simulink model "Single_Standalone_Module"  (R2019b)
settings: Solver=VariableStepAuto  StartTime=0.0  StopTime=1  RelTol=1e-3
libraries: powerlib x30, ac_grid_connnected x6, powerlib_meascontrol x4, Power_Electronic_Lab_Controllers x3, Control_Signal_Sources x1
settings Model: Creator=mehdi  LastModifiedBy=mehdi

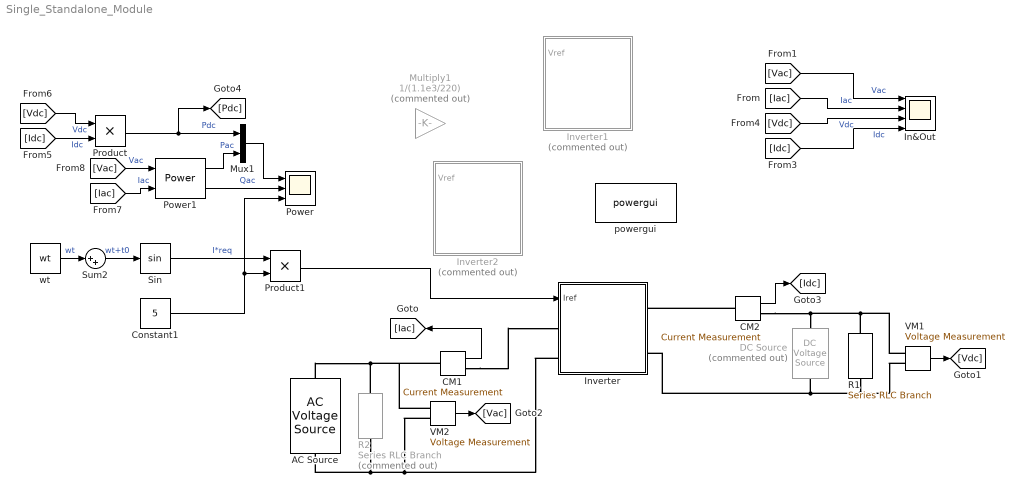
== system Single_Standalone_Module ==
  AC Source : powerlib/Electrical Sources/AC Voltage Source  Amplitude=220*sqrt(2)  Phase=0  Frequency=50  SampleTime=0  Measurements=None  BusType=swing  Pref=10e3  Qref=0  Qmin=-inf  Qmax=+inf
      settings: SourceProductName=Simscape Electrical
  CM1 : powerlib/Measurements/Current Measurement  PhasorSimulation=off  OutputType=Complex  PSBequivalent=0
      settings: SourceProductName=Simscape Electrical
  CM2 : powerlib/Measurements/Current Measurement  PhasorSimulation=off  OutputType=Complex  PSBequivalent=0
      settings: SourceProductName=Simscape Electrical
  Constant1 : Constant  Value=5
  DC Source : powerlib/Electrical Sources/DC Voltage Source  Commented=on  Amplitude=300  Measurements=None
      settings: SourceProductName=Simscape Electrical
  In&Out : Scope  NumInputPorts=4
  Inverter : Subsystem  mask{Pnom=1.1e3, Vnom=400, DC_Vol=600, DC_Cap=2*470e-6, is_cascaded=off, module=2, phase=3, f=50, fsw=10e3, mod_dom=[-1 1], mod_phs=90, input_type=Actaul, filter_type=LCL, L1=0.0089072, r1=0, Cf=1.0942e-06, Rf=42.5424, L2=0.0025465, r2=0, advance_designer=off, dVmax=0.05, dImax=0.5, des_type=dep. Ka, ka=0.1, r=0.1, fres=3419.0493, PR_P=0.1, PR_R=0.5, DC_Init=0, DC_Cap_ESR=0, start_time=0, PR_Scope_En=on, CG=1}
      mask prompts: Pnom "Nominal Power (W)"; Vnom "Nominal Voltage (V)"; DC_Vol "DC Link Voltage (V)"; DC_Cap "Capacitor (F)"; is_cascaded "Cascaded"; module "Number of modules in each phase"; phase "Number of Phases"; f "Found. Frequency (Hz)"; fsw "Switching Frequency (Hz)"; mod_dom "Modulator Domain [min MAX]"; mod_phs "Modulator Phase (Deg)"; input_type "Input Type"; filter_type "Filter Type"; L1 "Converter Side Ind (H)"; r1 "Converter Side Res (Ohm)"; Cf "Filter Capacitor (F)"; Rf "Filter Resistor (Ohm)"; L2 "Grid Side Ind (H)"; r2 "Grid Side Res (Ohm)"; advance_designer "Advance Designer"; dVmax "Max Accepted Voltage Variation"; dImax "Max Accepted Current Variation"; des_type "Designer Type"; fres "Resonant Freq."; PR_P "P"; PR_R "R"; DC_Init "DC Link Init (V)"; DC_Cap_ESR "DC Llink Cap ESR (Ohm)"; start_time "Start Time (s)"; PR_Scope_En "PR Controller Scope"; CG "Current Gain"
      mask Callback Pnom:
      | typ = get_param(gcb, 'input_type');
      | Pnom = str2num(get_param(gcb, 'Pnom'));
      | Vnom = str2num(get_param(gcb, 'Vnom'));
      | 
      | if strcmp(typ, 'Normalized')
      |     Inom = Pnom / Vnom ;
      |     set_param(gcb, 'CG', num2str(1 / Inom));
      | else
      |     set_param(gcb, 'CG', num2str(1));
      | end
      mask Callback Vnom:
      | typ = get_param(gcb, 'input_type');
      | Pnom = str2num(get_param(gcb, 'Pnom'));
      | Vnom = str2num(get_param(gcb, 'Vnom'));
      | 
      | if strcmp(typ, 'Normalized')
      |     Inom = Pnom / Vnom ;
      |     set_param(gcb, 'CG', num2str(1 / Inom));
      | else
      |     set_param(gcb, 'CG', num2str(1));
      | end
      mask Callback is_cascaded:
      | cas = get_param(gcb, 'is_cascaded');
      | mask = Simulink.Mask.get(gcb);
      | module = mask.getParameter('module');
      | phase  = mask.getParameter('phase');
      | 
      | if strcmp(cas, 'on')
      |     module.Visible = 'on';
      |     phase.Visible  = 'on';
      | 
      | else
      |     module.Visible = 'off';
      |     phase.Visible  = 'off';
      | 
      | end
      mask TypeOptions input_type: Actaul | Normalized
      mask Callback input_type:
      | typ = get_param(gcb, 'input_type');
      | Pnom = str2num(get_param(gcb, 'Pnom'));
      | Vnom = str2num(get_param(gcb, 'Vnom'));
      | 
      | if strcmp(typ, 'Normalized')
      |     Inom = Pnom / Vnom ;
      |     set_param(gcb, 'CG', num2str(1 / Inom));
      | else
      |     set_param(gcb, 'CG', num2str(1));
      | end
      mask TypeOptions filter_type: L | LC | LCL | LCL_imp
      mask Callback filter_type:
      | typ = get_param(gcb, 'filter_type');
      | mask = Simulink.Mask.get(gcb);
      | hL1 = mask.getParameter('L1');
      | hL2 = mask.getParameter('L2');
      | hCf = mask.getParameter('Cf');
      | hRf = mask.getParameter('Rf');
      | hr1 = mask.getParameter('r1');
      | hr2 = mask.getParameter('r2');
      | hKa = mask.getParameter('ka');
      | hR  = mask.getParameter('r');
      | hFr = mask.getParameter('fres');
      | hDT = mask.getParameter('des_type');
      | 
      | switch typ
      |     case 'L'
      |         hL2.Visible = 'off';
      |         hr2.Visible = 'off';
      |         hCf.Visible = 'off';
      |         hRf.Visible = 'off';
      |         hFr.Visible = 'off';
      |         hDT.Visible = 'off';
      |         hKa.Visible = 'off';
      |         hR.Visible  = 'off';
      | 
      |     case 'LC'
      |         hL2.Visible = 'off';
      |         hr2.Visible = 'off';
      |         hCf.Visible = 'on';
      |         hRf.Visible = 'on';
      |         hFr.Visible = 'on';
      |         hDT.Visible = 'off';
      |         hKa.Visible = 'off';
      |         hR.Visible  = 'off';
      | 
      |     case 'LCL'
      |         hL2.Visible = 'on';
      |         hr2.Visible = 'on';
      |         hCf.Visible = 'on';
      |         hRf.Visible = 'on';
      |         hFr.Visible = 'on';
      |         hDT.Visible = 'on';
      |         if strcmp(get_param(gcb, 'des_type'), 'dep. r')
      |             hR.Visible = 'on';
      |             hKa.Visible = 'off';
      |         else
      |             hR.Visible = 'off';
      |             hKa.Visible = 'on';
      |         end
      | end
      mask Callback advance_designer:
      | adv = get_param(gcb, 'advance_designer');
      | mask = Simulink.Mask.get(gcb);
      | dV = mask.getParameter('dVmax');
      | dI = mask.getParameter('dImax');
      | if strcmp(adv, 'on')
      |     dV.Visible = 'on';
      |     dI.Visible = 'on';
      | else
      |     dV.Visible = 'off';
      |     dI.Visible = 'off';
      | end
      mask TypeOptions des_type: dep. Ka | dep. r
      mask Callback des_type:
      | dep = get_param(gcb, 'des_type');
      | mask = Simulink.Mask.get(gcb);
      | ka = mask.getParameter('ka');
      | r  = mask.getParameter('r');
      | 
      | if strcmp(dep, 'dep. Ka')
      |     ka.Visible = 'on';
      |     r.Visible = 'off';
      | 
      | else
      |     ka.Visible = 'off';
      |     r.Visible = 'on';
      | 
      | end
      mask Callback PR_Scope_En:
      | enable = get_param(gcb, 'PR_Scope_En');
      | scope = getSimulinkBlockHandle(strjoin({gcb, 'PR'}, '/'));
      | 
      | if strcmp(enable, 'on')
      |     set(scope, 'Commented', 'off')
      | else
      |     set(scope, 'Commented', 'on')
      | end
      mask DialogControl Container7 Prompt: Basic
      mask DialogControl Container10 Prompt: Filter
      mask DialogControl Container16 Prompt: Filter Elements
      mask DialogControl cal Prompt: Calculator
      mask DialogControl cal Callback:
      | powericon('SinglePhaseLCLFIlterDesigner', 'calculator')
      | %powericon('ThreePhaseVSIwithLCL_CallBack', 'LCLFilterCalculator');
      mask DialogControl des Prompt: Designer
      mask DialogControl des Callback:
      | powericon('SinglePhaseLCLFIlterDesigner', 'desinger')
      | %powericon('ThreePhaseVSIwithLCL_CallBack', 'LCLFilterDesigner');
      mask DialogControl Container13 Prompt: Control & Simulation
      mask DialogControl Container14 Prompt: Control Parameters
      mask DialogControl Container17 Prompt: Initiat Values
      mask DialogControl Container18 Prompt: Simulation Controll
      mask DialogControl Container11 Prompt: Hidden Items
      mask Display: disp('Single\nPhase\nModule')
  Inverter1 : Subsystem  Commented=on  mask{Pnom=1.1e3, Vnom=230, DC_Vol=400, DC_Cap=470e-6, is_cascaded=off, module=2, phase=3, f=50, fsw=10e3, mod_dom=[-1 1], mod_phs=90, start_time=0, input_type=Actaul, L1=0.005914, L2=0.00084193, Cf=3.3095e-06, Rf=14.923, advance_designer=on, dVmax=0.05, dImax=0.5, des_type=dep. Ka, ka=0.1, r=0, fres=3222.5943, PR_P=0, PR_R=0}
      mask prompts: Pnom "Nominal Power (W)"; Vnom "Nominal Voltage (V)"; DC_Vol "DC Link Voltage (V)"; DC_Cap "Capacitor (F)"; is_cascaded "Cascaded"; module "Number of modules in each phase"; phase "Number of Phases"; f "Found. Frequency (Hz)"; fsw "Switching Frequency (Hz)"; mod_dom "Modulator Domain [min MAX]"; mod_phs "Modulator Phase (Deg)"; start_time "Start Time (s)"; input_type "Input Type"; L1 "Converter Side Ind (H)"; L2 "Grid Side Ind (H)"; Cf "Filter Capacitor (F)"; Rf "Filter Resistor (Ohm)"; advance_designer "Advance Designer"; dVmax "Max Accepted Voltage Variation"; dImax "Max Accepted Current Variation"; des_type "Designer Type"; fres "Resonant Freq."; PR_P "Prop Gain"; PR_R "Reso Gain"
      mask Callback is_cascaded:
      | cas = get_param(gcb, 'is_cascaded');
      | mask = Simulink.Mask.get(gcb);
      | module = mask.getParameter('module');
      | phase  = mask.getParameter('phase');
      | 
      | if strcmp(cas, 'on')
      |     module.Visible = 'on';
      |     phase.Visible  = 'on';
      | 
      | else
      |     module.Visible = 'off';
      |     phase.Visible  = 'off';
      | 
      | end
      mask TypeOptions input_type: Actaul | Normalized
      mask Callback advance_designer:
      | adv = get_param(gcb, 'advance_designer');
      | mask = Simulink.Mask.get(gcb);
      | dV = mask.getParameter('dVmax');
      | dI = mask.getParameter('dImax');
      | if strcmp(adv, 'on')
      |     dV.Visible = 'on';
      |     dI.Visible = 'on';
      | else
      |     dV.Visible = 'off';
      |     dI.Visible = 'off';
      | end
      mask TypeOptions des_type: dep. Ka | dep. r
      mask Callback des_type:
      | dep = get_param(gcb, 'des_type');
      | mask = Simulink.Mask.get(gcb);
      | ka = mask.getParameter('ka');
      | r  = mask.getParameter('r');
      | 
      | if strcmp(dep, 'dep. Ka')
      |     ka.Visible = 'on';
      |     r.Visible = 'off';
      | 
      | else
      |     ka.Visible = 'off';
      |     r.Visible = 'on';
      | 
      | end
      mask DialogControl Container7 Prompt: Basic
      mask DialogControl Container14 Prompt: Switching
      mask DialogControl Container10 Prompt: Filter
      mask DialogControl cal Prompt: Calculator
      mask DialogControl cal Callback: powericon('SinglePhaseLCLFIlterDesigner', 'calculator')
      mask DialogControl des Prompt: Designer
      mask DialogControl des Callback: powericon('SinglePhaseLCLFIlterDesigner', 'designer')
      mask DialogControl Container13 Prompt: Controller
      mask Display: disp('Inverter')
  Inverter2 : Subsystem  Commented=on  mask{Pnom=1.1e3, Vnom=230, DC_Vol=400, DC_Cap=470e-6, is_cascaded=on, module=2, phase=3, f=50, fsw=10e3, mod_dom=[-1 1], mod_phs=90, start_time=0, input_type=Actaul, L1=0.0089072, L2=0.00084193, Cf=3.3095e-06, Rf=11.7134, advance_designer=on, dVmax=0.05, dImax=0.5, des_type=dep. Ka, ka=0.1, r=0, fres=4105.6226, PR_P=0, PR_R=0, DC_Init=0, DC_Cap_ESR=0}
      mask prompts: Pnom "Nominal Power (W)"; Vnom "Nominal Voltage (V)"; DC_Vol "DC Link Voltage (V)"; DC_Cap "Capacitor (F)"; is_cascaded "Cascaded"; module "Number of modules in each phase"; phase "Number of Phases"; f "Found. Frequency (Hz)"; fsw "Switching Frequency (Hz)"; mod_dom "Modulator Domain [min MAX]"; mod_phs "Modulator Phase (Deg)"; start_time "Start Time (s)"; input_type "Input Type"; L1 "Converter Side Ind (H)"; L2 "Grid Side Ind (H)"; Cf "Filter Capacitor (F)"; Rf "Filter Resistor (Ohm)"; advance_designer "Advance Designer"; dVmax "Max Accepted Voltage Variation"; dImax "Max Accepted Current Variation"; des_type "Designer Type"; fres "Resonant Freq."; PR_P "Prop Gain"; PR_R "Reso Gain"; DC_Init "DC Link Init (V)"; DC_Cap_ESR "DC Llink Cap ESR (Ohm)"
      mask Callback is_cascaded:
      | cas = get_param(gcb, 'is_cascaded');
      | mask = Simulink.Mask.get(gcb);
      | module = mask.getParameter('module');
      | phase  = mask.getParameter('phase');
      | 
      | if strcmp(cas, 'on')
      |     module.Visible = 'on';
      |     phase.Visible  = 'on';
      | 
      | else
      |     module.Visible = 'off';
      |     phase.Visible  = 'off';
      | 
      | end
      mask TypeOptions input_type: Actaul | Normalized
      mask Callback advance_designer:
      | adv = get_param(gcb, 'advance_designer');
      | mask = Simulink.Mask.get(gcb);
      | dV = mask.getParameter('dVmax');
      | dI = mask.getParameter('dImax');
      | if strcmp(adv, 'on')
      |     dV.Visible = 'on';
      |     dI.Visible = 'on';
      | else
      |     dV.Visible = 'off';
      |     dI.Visible = 'off';
      | end
      mask TypeOptions des_type: dep. Ka | dep. r
      mask Callback des_type:
      | dep = get_param(gcb, 'des_type');
      | mask = Simulink.Mask.get(gcb);
      | ka = mask.getParameter('ka');
      | r  = mask.getParameter('r');
      | 
      | if strcmp(dep, 'dep. Ka')
      |     ka.Visible = 'on';
      |     r.Visible = 'off';
      | 
      | else
      |     ka.Visible = 'off';
      |     r.Visible = 'on';
      | 
      | end
      mask DialogControl Container7 Prompt: Basic
      mask DialogControl Container10 Prompt: Filter
      mask DialogControl cal Prompt: Calculator
      mask DialogControl cal Callback:
      | %powericon('SinglePhaseLCLFIlterDesigner', 'calculator')
      | powericon('ThreePhaseVSIwithLCL_CallBack', 'LCLFilterCalculator');
      mask DialogControl des Prompt: Designer
      mask DialogControl des Callback:
      | %powericon('SinglePhaseLCLFIlterDesigner', 'designer')
      | powericon('ThreePhaseVSIwithLCL_CallBack', 'LCLFilterDesigner');
      mask DialogControl Container13 Prompt: Controller
      mask Display: disp('Inverter')
  Multiply1 : Gain  Commented=on  Gain=1/(1.1e3/220)
  Mux1 : Mux  Inputs=2
  Power : Scope  NumInputPorts=3
  Power1 : powerlib_meascontrol/Measurements/Power  Freq=50  Vinit=[1, 0]  Iinit=[1, 0]  Ts=0
      settings: SourceProductName=Simscape Electrical
  Product : Product
  Product1 : Product
  R1 : powerlib/Elements/Series RLC Branch  LConnTagsString=__new0  RConnTagsString=__new0  BranchType=R  Resistance=82  Inductance=1e-3  SetiL0=off  InitialCurrent=0  Capacitance=1e-6  Setx0=off  InitialVoltage=0  Measurements=None
      settings: SourceProductName=Simscape Electrical
  R2 : powerlib/Elements/Series RLC Branch  Commented=on  LConnTagsString=__new0  RConnTagsString=__new0  BranchType=R  Resistance=40  Inductance=1e-3  SetiL0=off  InitialCurrent=0  Capacitance=1e-6  Setx0=off  InitialVoltage=0  Measurements=None
      settings: SourceProductName=Simscape Electrical
  Sin : Trigonometry
  Sum2 : Sum  Inputs=|++
  VM1 : powerlib/Measurements/Voltage Measurement  PhasorSimulation=off  OutputType=Complex  PSBequivalent=0
      settings: SourceProductName=Simscape Electrical
  VM2 : powerlib/Measurements/Voltage Measurement  PhasorSimulation=off  OutputType=Complex  PSBequivalent=0
      settings: SourceProductName=Simscape Electrical
  powergui : powerlib/powergui  Priority=1  SimulationMode=Continuous  SampleTime=50e-6  frequency=60  Iterations=50  frequencyindice=50  Pbase=100e6  ErrMax=1e-4  UnitsV=kV  UnitsW=MW  buscounter=0  FunctionMessages=off  echomessages=off  EnableUseOfTLC=off  CurrentSourceSwitches=off  DisableSnubberDevices=off  DisableRonSwitches=off  DisableVfSwitches=off  DisplayEquations=off  AutomaticDiscreteSolvers=off  SolverType=Tustin/Backward Euler (TBE)  Interpol=off  ExternalGateDelay=off  methode=off  Ts=100  x0status=blocks  SPID=on  SwTol=0  HookPort=off  NonlinearTolerance=1e-4  nMaxIteration=100  ContinueOnMaxIteration=off  RestoreLinks=warning  ResistiveCurrentMeasurement=off  Frange=[0:2:500]  Ylog=off  Xlog=on  ShowGrid=off  save=off  variable=ZData  structure=0  ZoomFFT=off  StartTime=0.0  cycles=1  DisplayStyle=1  fundamental=60  FreqAxis=off  MaxFrequency=1000  frequencyindicesteady=1  RmsSteady=1  display=off
      settings: SourceProductName=Simscape Electrical
  wt : Control_Signal_Sources/wt  f=100*pi  R=[-pi pi]
      settings: SourceProductName=Power Electronic Lab
  wires:
  CM1/1 -> [Iac]
  VM1/1 -> [Vdc]
  [Iac] -> In&Out/2  "Iac"
  VM2/1 -> [Vac]
  [Vac] -> In&Out/1  "Vac"
  CM2/1 -> [Idc]
  [Idc] -> In&Out/4  "Idc"
  [Vdc] -> In&Out/3  "Vdc"
  [Vdc] -> Product/1  "Vdc"
  [Idc] -> Product/2  "Idc"
  Sum2/1 -> Sin/1  "wt+t0"
  wt/1 -> Sum2/1  "wt"
  Power1/1 -> Mux1/2  "Pac"
  Mux1/1 -> Power/1
  [Vac] -> Power1/1  "Vac"
  [Iac] -> Power1/2  "Iac"
  Power1/2 -> Power/2  "Qac"
  Product/1 -> [Pdc], Mux1/1  "Pdc"
  Sin/1 -> Product1/1  "I*req"
  Product1/1 -> Inverter/1(Iref)
  Constant1/1 -> Product1/2, Power/3
  connections:
  R1/LConn1 -- VM1/LConn1 -- CM2/RConn1 -- DC Source/RConn1
  AC Source/RConn1 -- CM1/LConn1 -- VM2/LConn1 -- R2/LConn1
  VM2/LConn2 -- Inverter/LConn2 -- R2/RConn1 -- AC Source/LConn1
  VM1/LConn2 -- R1/RConn1 -- Inverter/RConn2 -- DC Source/LConn1
  CM2/LConn1 -- Inverter/RConn1
  CM1/RConn1 -- Inverter/LConn1

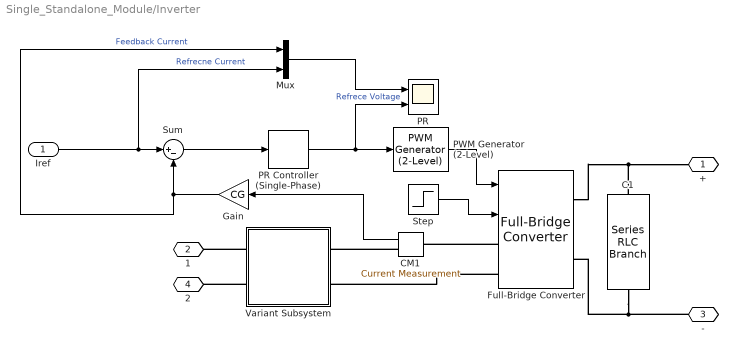
== system Single_Standalone_Module/Inverter ==
  Iref : Inport
  C1 : powerlib/Elements/Series RLC Branch  LConnTagsString=__new0  RConnTagsString=__new0  BranchType=RC  Resistance=DC_Cap_ESR  Inductance=0  SetiL0=off  InitialCurrent=0  Capacitance=DC_Cap  Setx0=on  InitialVoltage=DC_Init  Measurements=None
      settings: SourceProductName=Simscape Electrical
  CM1 : powerlib/Measurements/Current Measurement  PhasorSimulation=off  OutputType=Complex  PSBequivalent=0
      settings: SourceProductName=Simscape Electrical
  Full-Bridge Converter : powerlib/Power Electronics/Full-Bridge Converter  ModelType=Switching devices  Ron=1e-3  Rs=1e6  Cs=inf  Vforward=[0,0]  Ron_Diode=1e-3  Rs_Diode=1e6  Cs_Diode=inf  Vf_Diode=1e-3  Rs_CurrentSource=inf
      settings: SourceProductName=Simscape Electrical  SourceProductBaseCode=PS
  Gain : Gain  Gain=CG
  Mux : Mux  Inputs=2
  PR : Scope  NumInputPorts=2
  PR Controller (Single-Phase) : Power_Electronic_Lab_Controllers/PR Controller (Single-Phase)  Kp=PR_P  Kr=PR_R  w0=2*pi*f
      settings: SourceProductName=Power Electronic Lab
  PWM Generator (2-Level) : powerlib_meascontrol/Pulse & Signal Generators/PWM Generator (2-Level)  ModulatorType=Single-phase full-bridge (4 pulses)  ModulatorMode=Unsynchronized  Fc=fsw  Pc=mod_phs  nF=27  MinMax=mod_dom  SamplingTechnique=Natural  ModulatingSignals=off  m=0.8  Freq=60  Phase=0  Ts=0  ShowCarrierOutport=off
  Step : Step  Time=start_time  Before=1  After=0  SampleTime=0
  Sum : Sum  Inputs=|+-
  Variant Subsystem : Subsystem  VariantControlMode=Label  Variant=on  LabelModeActiveChoice=LCL_imp  mask{tp=filter_type, L1=L1, r1=r1, L2=L2, r2=r2, Cf=Cf, Rf=Rf}
      mask prompts: tp "Filter Type"
      mask Callback tp:
      | tp = get_param(gcb, 'tp');
      | 
      | switch tp
      |     case 'L'
      |         set_param(gcb, 'LabelModeActivechoice', 'L')
      | 
      |     case 'LC'
      |         set_param(gcb, 'LabelModeActivechoice', 'LC')
      | 
      |     case 'LCL'
      |         set_param(gcb, 'LabelModeActivechoice', 'LCL')
      | 
      |     case 'Devided LCL'
      |         set_param(gcb, 'LabelModeActivechoice', 'LCL_imp')
      | end
  + : PMIOPort  Side=Right
  1 : PMIOPort  Port=2  Side=Left
  - : PMIOPort  Port=3  Side=Right
  2 : PMIOPort  Port=4  Side=Left
  wires:
  PWM Generator (2-Level)/1 -> Full-Bridge Converter/1
  Step/1 -> Full-Bridge Converter/2
  Sum/1 -> PR Controller (Single-Phase)/1
  PR Controller (Single-Phase)/1 -> PR/2, PWM Generator (2-Level)/1  "Refrece Voltage"
  Iref/1 -> Mux/2, Sum/1  "Refrecne Current"
  Mux/1 -> PR/1
  Gain/1 -> Mux/1, Sum/2  "Feedback Current"
  CM1/1 -> Gain/1
  connections:
  Full-Bridge Converter/RConn1 -- C1/LConn1 -- +/RConn1
  -/RConn1 -- C1/RConn1 -- Full-Bridge Converter/RConn2
  Variant Subsystem/RConn2 -- 2/RConn1
  Full-Bridge Converter/LConn2 -- Variant Subsystem/LConn2
  Full-Bridge Converter/LConn1 -- CM1/LConn1
  CM1/RConn1 -- Variant Subsystem/LConn1
  Variant Subsystem/RConn1 -- 1/RConn1

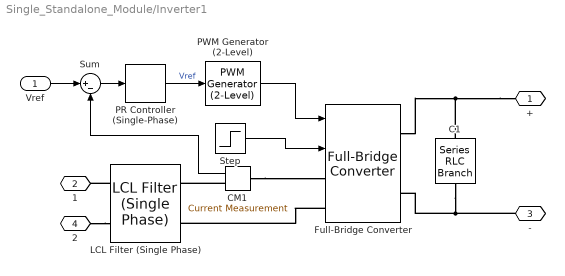
== system Single_Standalone_Module/Inverter1 ==
  Vref : Inport
  C1 : powerlib/Elements/Series RLC Branch  LConnTagsString=__new0  RConnTagsString=__new0  BranchType=C  Resistance=40  Inductance=1e-3  SetiL0=off  InitialCurrent=0  Capacitance=470e-6  Setx0=off  InitialVoltage=0  Measurements=None
      settings: SourceProductName=Simscape Electrical
  CM1 : powerlib/Measurements/Current Measurement  PhasorSimulation=off  OutputType=Complex  PSBequivalent=0
      settings: SourceProductName=Simscape Electrical
  Full-Bridge Converter : powerlib/Power Electronics/Full-Bridge Converter  ModelType=Switching devices  Ron=1e-3  Rs=1e6  Cs=inf  Vforward=[0,0]  Ron_Diode=1e-3  Rs_Diode=1e6  Cs_Diode=inf  Vf_Diode=1e-3  Rs_CurrentSource=inf
      settings: SourceProductName=Simscape Electrical  SourceProductBaseCode=PS
  LCL Filter (Single Phase) : ac_grid_connnected/LCL Filter (Single Phase)  Vn=400  Vdc=600  Sn=1.1e3  f=50  fsw=10e3  L1=0.0089072  L2=0.0025465  Cf=1.0942e-06  Rf=42.5424  advance_designer_ckb=on  dVmax=0.05  dImax=0.5  des_pop=known ka  ka=0.1  r=0  fres=3419.0493
      settings: SourceProductName=Power Electronic Lab
  PR Controller (Single-Phase) : Power_Electronic_Lab_Controllers/PR Controller (Single-Phase)  Kp=0.1  Kr=0.5  w0=100*pi
      settings: SourceProductName=Power Electronic Lab
  PWM Generator (2-Level) : powerlib_meascontrol/Pulse & Signal Generators/PWM Generator (2-Level)  ModulatorType=Single-phase full-bridge (4 pulses)  ModulatorMode=Unsynchronized  Fc=10e3  Pc=90  nF=27  MinMax="[ -1  1 ]"  SamplingTechnique=Natural  ModulatingSignals=off  m=0.8  Freq=60  Phase=0  Ts=0  ShowCarrierOutport=off
  Step : Step  Time=0  Before=1  After=0  SampleTime=0
  Sum : Sum  Inputs=|+-
  + : PMIOPort  Side=Right
  1 : PMIOPort  Port=2  Side=Left
  - : PMIOPort  Port=3  Side=Right
  2 : PMIOPort  Port=4  Side=Left
  wires:
  CM1/1 -> Sum/2
  Vref/1 -> Sum/1
  PR Controller (Single-Phase)/1 -> PWM Generator (2-Level)/1  "Vref"
  Sum/1 -> PR Controller (Single-Phase)/1
  Step/1 -> Full-Bridge Converter/2
  PWM Generator (2-Level)/1 -> Full-Bridge Converter/1
  connections:
  CM1/RConn1 -- LCL Filter (Single Phase)/LConn1
  CM1/LConn1 -- Full-Bridge Converter/LConn1
  Full-Bridge Converter/RConn2 -- C1/RConn1 -- -/RConn1
  +/RConn1 -- C1/LConn1 -- Full-Bridge Converter/RConn1
  Full-Bridge Converter/LConn2 -- LCL Filter (Single Phase)/LConn2
  2/RConn1 -- LCL Filter (Single Phase)/RConn2
  LCL Filter (Single Phase)/RConn1 -- 1/RConn1

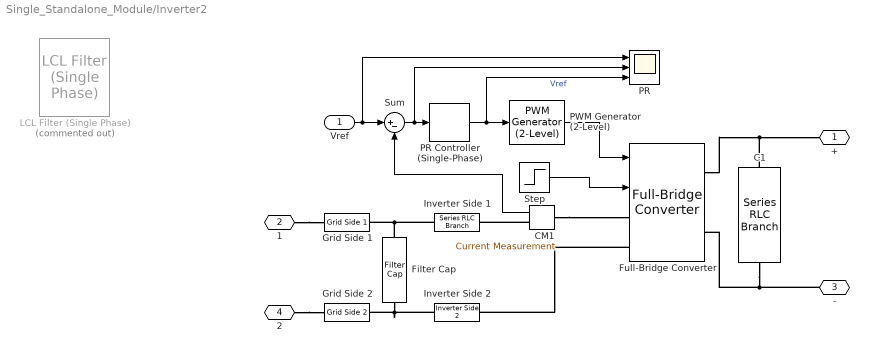
== system Single_Standalone_Module/Inverter2 ==
  Vref : Inport
  C1 : powerlib/Elements/Series RLC Branch  LConnTagsString=__new0  RConnTagsString=__new0  BranchType=RC  Resistance=DC_Cap_ESR  Inductance=0  SetiL0=off  InitialCurrent=0  Capacitance=DC_Cap  Setx0=on  InitialVoltage=DC_Init  Measurements=None
      settings: SourceProductName=Simscape Electrical
  CM1 : powerlib/Measurements/Current Measurement  PhasorSimulation=off  OutputType=Complex  PSBequivalent=0
      settings: SourceProductName=Simscape Electrical
  Filter Cap : ac_grid_connnected/LCL Filter (Single Phase)/Filter Cap  LConnTagsString=__new0  RConnTagsString=__new0  BranchType=RC  Resistance=Rf  Inductance=L2  SetiL0=off  InitialCurrent=0  Capacitance=Cf  Setx0=off  InitialVoltage=0  Measurements=None
      settings: SourceProductName=Power Electronic Lab
  Full-Bridge Converter : powerlib/Power Electronics/Full-Bridge Converter  ModelType=Switching devices  Ron=1e-3  Rs=1e6  Cs=inf  Vforward=[0,0]  Ron_Diode=1e-3  Rs_Diode=1e6  Cs_Diode=inf  Vf_Diode=1e-3  Rs_CurrentSource=inf
      settings: SourceProductName=Simscape Electrical  SourceProductBaseCode=PS
  Grid Side 1 : ac_grid_connnected/LCL Filter (Single Phase)/Grid Side 1  LConnTagsString=__new0  RConnTagsString=__new0  BranchType=L  Resistance=1  Inductance=L2/2  SetiL0=off  InitialCurrent=0  Capacitance=1e-6  Setx0=off  InitialVoltage=0  Measurements=None
      settings: SourceProductName=Power Electronic Lab
  Grid Side 2 : ac_grid_connnected/LCL Filter (Single Phase)/Grid Side 2  LConnTagsString=__new0  RConnTagsString=__new0  BranchType=L  Resistance=1  Inductance=L2/2  SetiL0=off  InitialCurrent=0  Capacitance=1e-6  Setx0=off  InitialVoltage=0  Measurements=None
      settings: SourceProductName=Power Electronic Lab
  Inverter Side 1 : powerlib/Elements/Series RLC Branch  LConnTagsString=__new0  RConnTagsString=__new0  BranchType=L  Resistance=1  Inductance=L1/2  SetiL0=off  InitialCurrent=0  Capacitance=1e-6  Setx0=off  InitialVoltage=0  Measurements=None
      settings: SourceProductName=Simscape Electrical
  Inverter Side 2 : ac_grid_connnected/LCL Filter (Single Phase)/Inverter Side 2  LConnTagsString=__new0  RConnTagsString=__new0  BranchType=L  Resistance=1  Inductance=L1/2  SetiL0=off  InitialCurrent=0  Capacitance=1e-6  Setx0=off  InitialVoltage=0  Measurements=None
      settings: SourceProductName=Power Electronic Lab
  LCL Filter (Single Phase) : ac_grid_connnected/LCL Filter (Single Phase)  Commented=on  Vn=400  Vdc=600  Sn=1.1e3  f=50  fsw=10e3  L1=L1  L2=L2  Cf=Cf  Rf=Rf  advance_designer_ckb=on  dVmax=0.05  dImax=0.5  des_pop=known ka  ka=0.1  r=0  fres=3419.0493
      settings: SourceProductName=Power Electronic Lab
  PR : Scope  NumInputPorts=3
  PR Controller (Single-Phase) : Power_Electronic_Lab_Controllers/PR Controller (Single-Phase)  Kp=0.1  Kr=0.5  w0=100*pi
      settings: SourceProductName=Power Electronic Lab
  PWM Generator (2-Level) : powerlib_meascontrol/Pulse & Signal Generators/PWM Generator (2-Level)  ModulatorType=Single-phase full-bridge (4 pulses)  ModulatorMode=Unsynchronized  Fc=fsw  Pc=mod_phs  nF=27  MinMax=mod_dom  SamplingTechnique=Natural  ModulatingSignals=off  m=0.8  Freq=60  Phase=0  Ts=0  ShowCarrierOutport=off
  Step : Step  Time=start_time  Before=1  After=0  SampleTime=0
  Sum : Sum  Inputs=|+-
  + : PMIOPort  Side=Right
  1 : PMIOPort  Port=2  Side=Left
  - : PMIOPort  Port=3  Side=Right
  2 : PMIOPort  Port=4  Side=Left
  wires:
  CM1/1 -> Sum/2
  Vref/1 -> Sum/1, PR/1
  PR Controller (Single-Phase)/1 -> PWM Generator (2-Level)/1, PR/3  "Vref"
  Sum/1 -> PR Controller (Single-Phase)/1, PR/2
  Step/1 -> Full-Bridge Converter/2
  PWM Generator (2-Level)/1 -> Full-Bridge Converter/1
  connections:
  Full-Bridge Converter/LConn2 -- Inverter Side 2/RConn1
  CM1/RConn1 -- Inverter Side 1/LConn1
  Grid Side 2/RConn1 -- Filter Cap/RConn1 -- Inverter Side 2/LConn1
  Grid Side 1/LConn1 -- Filter Cap/LConn1 -- Inverter Side 1/RConn1
  1/RConn1 -- Grid Side 1/RConn1
  2/RConn1 -- Grid Side 2/LConn1
  CM1/LConn1 -- Full-Bridge Converter/LConn1
  Full-Bridge Converter/RConn2 -- C1/RConn1 -- -/RConn1
  C1/LConn1 -- Full-Bridge Converter/RConn1 -- +/RConn1

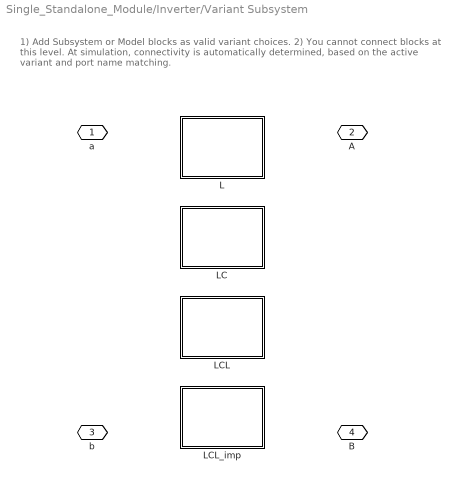
== system Single_Standalone_Module/Inverter/Variant Subsystem ==
  note: 1) Add Subsystem or Model blocks as valid variant choices.
      | 2) You cannot connect blocks at this level. At simulation, connectivity is automatically
      | determined, based on the active variant and port name matching.
  L : Subsystem  VariantControl=L
  LC : Subsystem  VariantControl=LC
  LCL : Subsystem  VariantControl=LCL
  LCL_imp : Subsystem  VariantControl=LCL_imp
  a : PMIOPort  Side=Right
  A : PMIOPort  Port=2  Side=Left
  b : PMIOPort  Port=3  Side=Right
  B : PMIOPort  Port=4  Side=Left

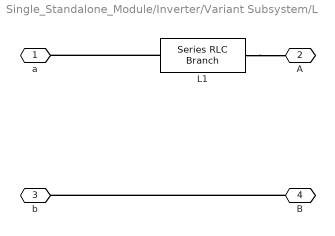
== system Single_Standalone_Module/Inverter/Variant Subsystem/L ==
  L1 : powerlib/Elements/Series RLC Branch  LConnTagsString=__new0  RConnTagsString=__new0  BranchType=RL  Resistance=r1  Inductance=L1  SetiL0=off  InitialCurrent=0  Capacitance=1e-6  Setx0=off  InitialVoltage=0  Measurements=None
      settings: SourceProductName=Simscape Electrical
  a : PMIOPort  Side=Right
  A : PMIOPort  Port=2  Side=Left
  b : PMIOPort  Port=3  Side=Right
  B : PMIOPort  Port=4  Side=Left
  connections:
  B/RConn1 -- b/RConn1
  L1/RConn1 -- a/RConn1
  L1/LConn1 -- A/RConn1

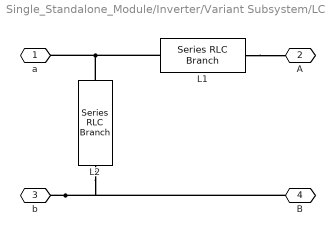
== system Single_Standalone_Module/Inverter/Variant Subsystem/LC ==
  L1 : powerlib/Elements/Series RLC Branch  LConnTagsString=__new0  RConnTagsString=__new0  BranchType=RL  Resistance=r1  Inductance=L1  SetiL0=off  InitialCurrent=0  Capacitance=1e-6  Setx0=off  InitialVoltage=0  Measurements=None
      settings: SourceProductName=Simscape Electrical
  L2 : powerlib/Elements/Series RLC Branch  LConnTagsString=__new0  RConnTagsString=__new0  BranchType=RC  Resistance=Rf  Inductance=L1  SetiL0=off  InitialCurrent=0  Capacitance=Cf  Setx0=off  InitialVoltage=0  Measurements=None
      settings: SourceProductName=Simscape Electrical
  a : PMIOPort  Side=Right
  A : PMIOPort  Port=2  Side=Left
  b : PMIOPort  Port=3  Side=Right
  B : PMIOPort  Port=4  Side=Left
  connections:
  L1/LConn1 -- A/RConn1
  L2/LConn1 -- L1/RConn1 -- a/RConn1
  b/RConn1 -- L2/RConn1 -- B/RConn1

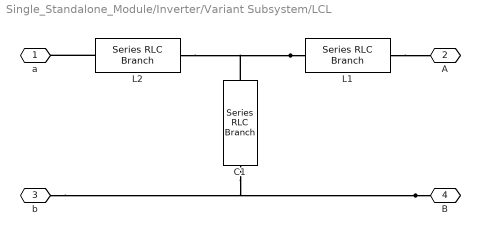
== system Single_Standalone_Module/Inverter/Variant Subsystem/LCL ==
  C1 : powerlib/Elements/Series RLC Branch  LConnTagsString=__new0  RConnTagsString=__new0  BranchType=RC  Resistance=Rf  Inductance=L1  SetiL0=off  InitialCurrent=0  Capacitance=Cf  Setx0=off  InitialVoltage=0  Measurements=None
      settings: SourceProductName=Simscape Electrical
  L1 : powerlib/Elements/Series RLC Branch  LConnTagsString=__new0  RConnTagsString=__new0  BranchType=RL  Resistance=r1  Inductance=L1  SetiL0=off  InitialCurrent=0  Capacitance=1e-6  Setx0=off  InitialVoltage=0  Measurements=None
      settings: SourceProductName=Simscape Electrical
  L2 : powerlib/Elements/Series RLC Branch  LConnTagsString=__new0  RConnTagsString=__new0  BranchType=RL  Resistance=r2  Inductance=L2  SetiL0=off  InitialCurrent=0  Capacitance=1e-6  Setx0=off  InitialVoltage=0  Measurements=None
      settings: SourceProductName=Simscape Electrical
  a : PMIOPort  Side=Right
  A : PMIOPort  Port=2  Side=Left
  b : PMIOPort  Port=3  Side=Right
  B : PMIOPort  Port=4  Side=Left
  connections:
  B/RConn1 -- C1/RConn1 -- b/RConn1
  L1/RConn1 -- C1/LConn1 -- L2/LConn1
  L1/LConn1 -- A/RConn1
  L2/RConn1 -- a/RConn1

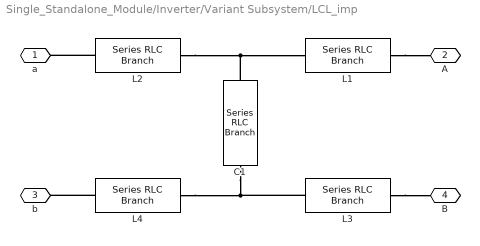
== system Single_Standalone_Module/Inverter/Variant Subsystem/LCL_imp ==
  C1 : powerlib/Elements/Series RLC Branch  LConnTagsString=__new0  RConnTagsString=__new0  BranchType=RC  Resistance=Rf  Inductance=L1  SetiL0=off  InitialCurrent=0  Capacitance=Cf  Setx0=off  InitialVoltage=0  Measurements=None
      settings: SourceProductName=Simscape Electrical
  L1 : powerlib/Elements/Series RLC Branch  LConnTagsString=__new0  RConnTagsString=__new0  BranchType=RL  Resistance=r1/2  Inductance=L1/2  SetiL0=off  InitialCurrent=0  Capacitance=1e-6  Setx0=off  InitialVoltage=0  Measurements=None
      settings: SourceProductName=Simscape Electrical
  L2 : powerlib/Elements/Series RLC Branch  LConnTagsString=__new0  RConnTagsString=__new0  BranchType=RL  Resistance=r2/2  Inductance=L2/2  SetiL0=off  InitialCurrent=0  Capacitance=1e-6  Setx0=off  InitialVoltage=0  Measurements=None
      settings: SourceProductName=Simscape Electrical
  L3 : powerlib/Elements/Series RLC Branch  LConnTagsString=__new0  RConnTagsString=__new0  BranchType=RL  Resistance=r1/2  Inductance=L1/2  SetiL0=off  InitialCurrent=0  Capacitance=1e-6  Setx0=off  InitialVoltage=0  Measurements=None
      settings: SourceProductName=Simscape Electrical
  L4 : powerlib/Elements/Series RLC Branch  LConnTagsString=__new0  RConnTagsString=__new0  BranchType=RL  Resistance=r2/2  Inductance=L2/2  SetiL0=off  InitialCurrent=0  Capacitance=1e-6  Setx0=off  InitialVoltage=0  Measurements=None
      settings: SourceProductName=Simscape Electrical
  a : PMIOPort  Side=Right
  A : PMIOPort  Port=2  Side=Left
  b : PMIOPort  Port=3  Side=Right
  B : PMIOPort  Port=4  Side=Left
  connections:
  L2/RConn1 -- a/RConn1
  L1/LConn1 -- A/RConn1
  L2/LConn1 -- C1/LConn1 -- L1/RConn1
  L3/LConn1 -- C1/RConn1 -- L4/RConn1
  L3/RConn1 -- B/RConn1
  L4/LConn1 -- b/RConn1
